simulink model "Resampler_Stream_Ex2"  (R2023a)
settings: Solver=VariableStepAuto  StartTime=0.0  StopTime=2  RelTol=1e-3
undefined symbols (not defined in the file): designMultirateFIR, None, S, vsva2197, xcvc1902
libraries: aieDSP x1, dspsrcs4 x1, dspmlti4 x1, vmcUtilities x1
settings Model: Creator=sdegala  LastModifiedBy=robg
settings ModelReferenceCC: EnableRefExpFcnMdlSchedulingChecks=on

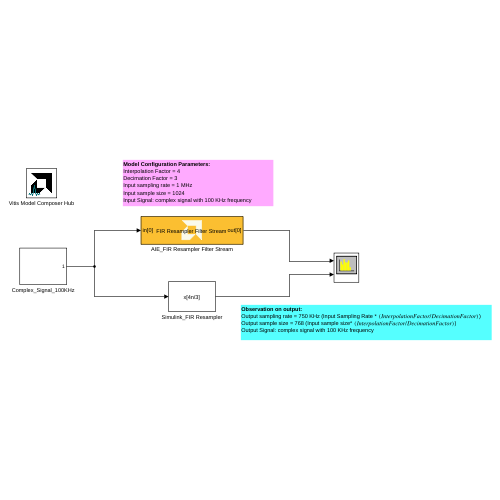
[thumbnail: Simulink's stored preview of the top-level diagram]
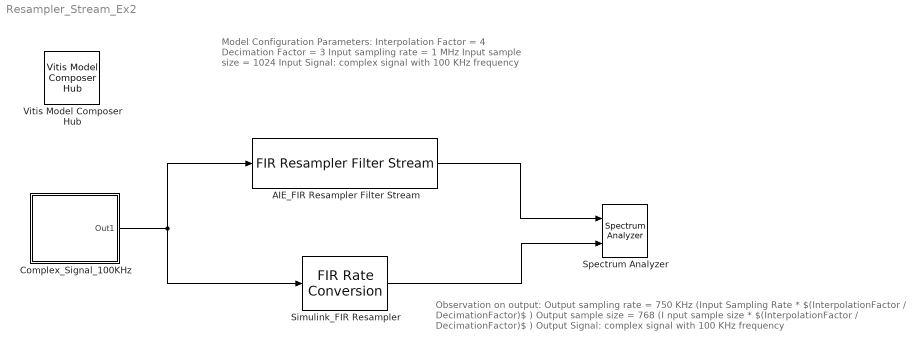
== system Resampler_Stream_Ex2 ==
  note: Model Configuration Parameters:
      | Interpolation Factor = 4
      | Decimation Factor = 3
      | Input sampling rate = 1 MHz
      | Input sample size = 1024
      | Input Signal: complex signal with 100 KHz frequency
  note: Observation on output:
      | Output sampling rate = 750 KHz (Input Sampling Rate * $(InterpolationFactor / DecimationFactor)$ )
      | Output sample size = 768 (I nput sample size * $(InterpolationFactor / DecimationFactor)$ )
      | Output Signal: complex signal with 100 KHz frequency
  AIE_FIR Resampler Filter Stream : aieDSP/FIR Resampler Filter Stream  data_type=cfloat  coef_type=float  use_coeff_reload=off  dual_ip=off  num_outputs=off  coeff=designMultirateFIR(3,4)  fir_length=30  interpolate_factor=3  decimate_factor=4  input_window_size=1024  shift_val=0  rnd_mode=Round to positive infinity  sat_mode=0-None  ssr=1  interp_poly=1  deci_poly=1  casc_length=4  AIE_VARIANT=1  blockJsonConstraints=[]  blockJsonConstraintsInternal=[]  spec=vmc_stream_fir_resampler.json  SerializedMaskParamNames=[]  SerializedMaskParamValues=[]  SerializedMaskParamVisibilities=[]  block_type=FIR Resampler Filter Stream  SerializedMaskParamDataypes=typename|typename|bool|bool|bool|coef_type|uint|uint|uint|uint|uint|uint|uint|uint|uint|uint|uint|uint  SerializedMaskParamEnumStrArr=0|0|0|0|0|0|0|0|0|0|0|Floor,Ceiling,Round to positive infinity,Round to negative infinity,Round symmetrical to infinity,Round symmetrical to zero,Round convergent to even,Round convergent to odd|0-None,1-Asymmetric,3-Symmetric|0|0|0|0|0  SerializedMaskParamEnumValArr=0|0|0|0|0|0|0|0|0|0|0|0,1,2,3,4,5,6,7|0,1,3|0|0|0|0|0  SerializedMaskParamVectorArr=0|0|0|0|0|1|0|0|0|0|0|0|0|0|0|0|0|0
  Complex_Signal_100KHz : Subsystem
  Simulink_FIR Resampler : dspmlti4/FIR Rate Conversion  FilterSource=Dialog parameters  L=3  h=designMultirateFIR(3,4)  M=4  FilterObject=FRC  rateMode=Enforce single-rate processing  AllowArbitraryInputLength=off  roundingMode=Floor  overflowMode=off  firstCoeffDataTypeStr=Inherit: Same word length as input  firstCoeffMin=[]  firstCoeffMax=[]  firstCoeffLastDataTypeStr=Inherit: Same word length as input  outputDataTypeStr=Inherit: Same as accumulator  outputMin=[]  outputMax=[]  outputLastDataTypeStr=Inherit: Same as accumulator
  Spectrum Analyzer : SpectrumAnalyzer  NumInputPorts=2  AveragingMethod=Exponential  Title=AIE and Simulink Resampler stream block comparison  ShowLegend=on  ChannelNames="[\"\"]"  DefaultConfigurationName=spbscopes.SpectrumAnalyzerBlockCfg
  Vitis Model Composer Hub : vmcUtilities/Vitis Model Composer Hub  Tag=genX  CodeGeneration=off  StartColumn=1  NumberOfColumns=1  TargetDirectory=./code  exportDesign=off  analyzeDesign=off  validateDesignOnHw=off  ExportType=AI Engines  IpVendor=xilinx.com  IpLibrary=hls  IpVersion=1.0  IpHWLanguage=Verilog  AieCompilerOptions={}  AieSimulatorOptions={}  CreateTestbench=off  TestbenchStackSize=10  RunRtlSim=off  RunCSim=off  RunAieSim=off  AieSimTimeout=50000  RunAieSimProfiling=off  LaunchVitisAnalyzer=off  PlotOutput=off  RunX86Sim=off  X86SimTimeout=10  GenHwImage=off  GenLibadfXo=off  GenHwValidationCode=off  PlatformType=Not Specified  HwSystemType=Baremetal  HwValidationTarget=hw  ProjDevice=xcvc1902-vsva2197-1LP-e-S  ProjDevicePart=xcvc1902-vsva2197-1LP-e-S  AIEType=AIE  SamplePeriod=-1  ClockFrequency=200  DataPathParallelism=1  xilinxfamily=versalaicore  part=xcvc1902  speed=-1LP-e-S  package=vsva2197  directory=./netlist  testbench=off  incr_netlist=off  synthesis_tool=Vivado  clock_wrapper=Clock Enables  dbl_ovrd=According to Block Masks  dcm_input_clock_period=10  sysclk_period=10  simulink_period=1  eval_field=0  LogFileName=''  NThreads=4
  wires:
  Simulink_FIR Resampler/1 -> Spectrum Analyzer/2
  AIE_FIR Resampler Filter Stream/1 -> Spectrum Analyzer/1
  Complex_Signal_100KHz/1(Out1) -> AIE_FIR Resampler Filter Stream/1, Simulink_FIR Resampler/1

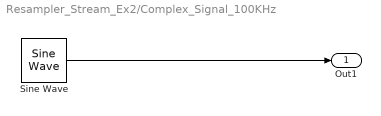
== system Resampler_Stream_Ex2/Complex_Signal_100KHz ==
  Sine Wave : dspsrcs4/Sine Wave  Amplitude=1  Frequency=100e3  Phase=0  SampleMode=Discrete  OutComplex=Complex  CompMethod=Trigonometric fcn  TableSize=Speed  SampleTime=1/1e6  SamplesPerFrame=1024  ResetState=Restart at time zero  OutputFrames=off  dataType=single  wordLen=16  udDataType=sfix(16)  fracBitsMode=Best precision  numFracBits=15  OutDataTypeStr=single  LastOutDataTypeStr=single
  Out1 : Outport
  wires:
  Sine Wave/1 -> Out1/1
